simulink model "inner_PD_thrust_d"  (R2016a)
settings: Solver=VariableStepAuto  StartTime=0.0  StopTime=10  RelTol=1e-3

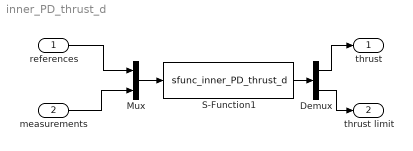
== system inner_PD_thrust_d ==
  references : Inport  PortDimensions=12
  measurements : Inport  Port=2  PortDimensions=12
  Demux : Demux  Outputs=2
  Mux : Mux  Inputs=2
  S-Function1 : S-Function  FunctionName=sfunc_inner_PD_thrust_d  Parameters=PD_thrust_param  SFunctionDeploymentMode=off  EnableBusSupport=off
  thrust : Outport
  thrust limit : Outport  Port=2
  wires:
  measurements/1 -> Mux/2
  references/1 -> Mux/1
  Mux/1 -> S-Function1/1
  S-Function1/1 -> Demux/1
  Demux/1 -> thrust/1
  Demux/2 -> thrust limit/1
